simulink subsystem "wheel_dyn"  (R2022a)
settings: Solver=VariableStepAuto  StartTime=0.0  StopTime=10.0  RelTol=1e-3
libraries: dspinverses x1
settings Model: Creator=samuel  LastModifiedBy=samuel

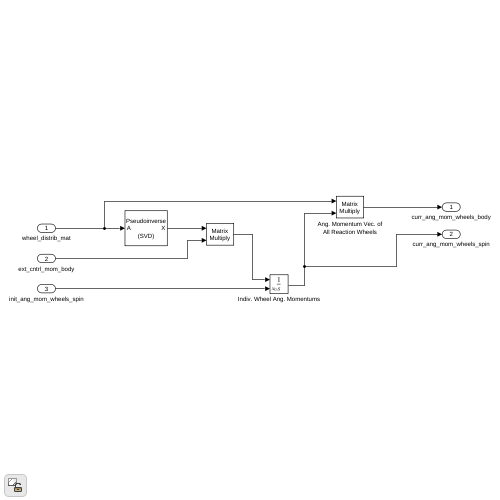
[thumbnail: Simulink's stored preview of the top-level diagram]
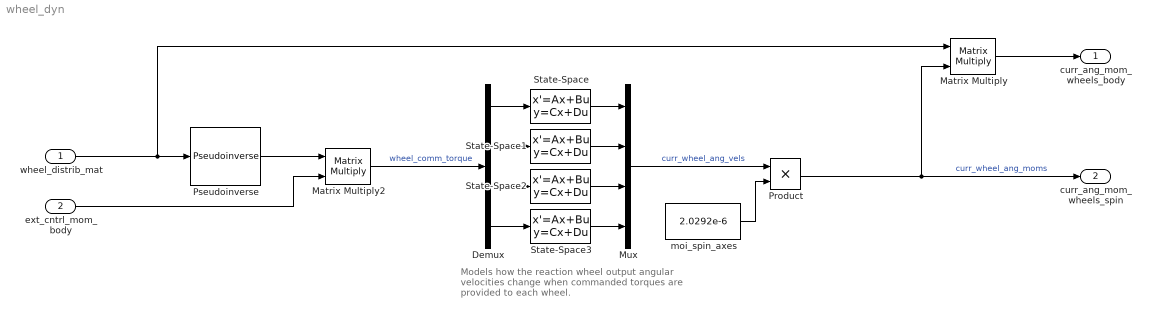
== system wheel_dyn ==
  note: Models how the reaction wheel output angular velocities change when commanded torques are provided to each wheel.
  wheel_distrib_mat : Inport
  ext_cntrl_mom_body : Inport  Port=2
  Demux : Demux
  Matrix Multiply : Product  Multiplication=Matrix(*)
  Matrix Multiply2 : Product  Multiplication=Matrix(*)
  Mux : Mux
  Product : Product
  Pseudoinverse : dspinverses/Pseudoinverse  wanterr=off  SimulateUsing=Interpreted execution
      settings: SourceProductBaseCode=DS
  State-Space{,1..3} (4 alike) : StateSpace  A=-0.02216  B=512  C=962.5  D=0  InitialCondition=0  ParameterTunability=Unconstrained
  moi_spin_axes : Constant  Value=2.0292e-6
  curr_ang_mom_wheels_body : Outport
  curr_ang_mom_wheels_spin : Outport  Port=2
  wires:
  Pseudoinverse/1 -> Matrix Multiply2/1
  ext_cntrl_mom_body/1 -> Matrix Multiply2/2
  Matrix Multiply2/1 -> Demux/1  "wheel_comm_torque"
  wheel_distrib_mat/1 -> Pseudoinverse/1, Matrix Multiply/1
  Matrix Multiply/1 -> curr_ang_mom_wheels_body/1
  Product/1 -> Matrix Multiply/2, curr_ang_mom_wheels_spin/1  "curr_wheel_ang_moms"
  Demux/1 -> State-Space/1
  Demux/2 -> State-Space1/1
  Demux/3 -> State-Space2/1
  Demux/4 -> State-Space3/1
  State-Space/1 -> Mux/1
  State-Space1/1 -> Mux/2
  State-Space2/1 -> Mux/3
  State-Space3/1 -> Mux/4
  Mux/1 -> Product/1  "curr_wheel_ang_vels"
  moi_spin_axes/1 -> Product/2
